simulink model "NarmaMotorS555"  (R2019b)
settings: Solver=FixedStepAuto  StartTime=0.0  StopTime=30  FixedStep=0.001  RelTol=1e-3
libraries: neural x1, simulink x1
settings Model: Creator=Emanuel  LastModifiedBy=Emanuel

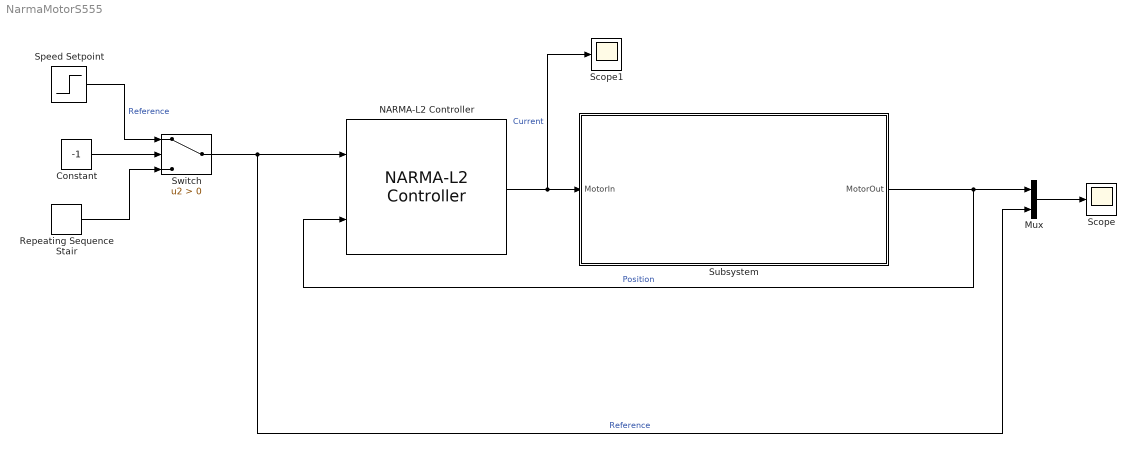
== system NarmaMotorS555 ==
  Constant : Constant  Value=-1
  Mux : Mux  Inputs=2
  NARMA-L2 Controller : neural/Control Systems/NARMA-L2 Controller  Normalize=0  IW1_1=[21.420472575406133586 -21.972703296207392043 -7.9906893081249545929 7.0093970032024079941 8.5373540872644628763 8.8150101640927438496 -2.9213191886093334837 -1.6299775720800899759 -1.2105815169084979122;-0.12814212482981091057 -15.451137614433791967 23.631470507291648886 8.1296696368918119902 -15.652038067620965833 46.375391110128518335 -18.123857574027180561 2.2201217276273146339 -5.7721001387385229009;0.00011021763309481335483 -2.9231777266735832472e-05 1.0017262420479688574e-05 4.4951441027179193515e-06 -1.3997667040411272311e-05 0.00015970236645007296014 -1.3053492369251622356e-05 -0.00010774931406669859316 -0.00020601444658894911294;-10.80852230598250685 2.9694610081311818561 23.641173482018462693 -8.9374523387581881195 -6.2415329671022758973 -12.804217284426561818 8.9963311782389041582 6.791537241510962275 -12.300046900155798824;-2.5462998703491250829 0.40736130073714715838 -18.235100932779950256 1.6768821975697136839 20.314826651060510443 8.341267777448827303 31.645810426981082486 20.102565537518792382 -8.4636642447471075457]  IW3_2=[26.518110030274044675 11.942738916641486568 5.9317929528543604789 -12.906642684649902719 -35.475911845893101315 -0.11447224640092470982 1.1036063891538443471 1.2539998649502879235 1.9551365056904561612;-39.675892314256245186 -12.346459002706955843 12.885795078472623842 15.915516809313654534 24.244911915898089916 -3.9565933976663298921 -13.490028317496282284 -1.9222873594971927602 1.9450222464410471535;-0.49775896817409004402 -20.203686361997281296 15.185910851212808481 6.5982122964106935115 -3.3039127819307578804 5.661531661101603774 1.0333906568373585344 3.2167073441307101334 2.3975065135655868609;-18.741605900013510677 17.739672652356080818 -8.5348038689952723246 -1.7678605588439249008 10.151016666991511173 6.010383209140059968 3.0879575435889647927 6.4865290493294747165 -2.8848587536067671344;9.4392585237701105427 8.6634826964493463208 5.7064818124290734858 4.3740389144362650242 4.6910020487183228255 0.25543532051108375214 0.37978770358499319704 0.25144757086620406206 -0.19880708237697139462]  IW5_3=-3.3096476108531893701  LW2_1=[-33.532867616268568156 -0.062278984235911556688 -126.85135625090671851 -0.22775640561207807777 0.011587551941983549944]  LW4_3=[-0.12271840530871241937 0.019979545310268350539 3.9480102969725656692 -3.8012667565729301167 -4.8370809941710657398]  LW5_4=0.32653514050989068673  LW6_5=0.51420792674405046974  LW6_2=-96.852303453609138728  B1=[2.427680381206728466;-3.6329489870410958119;-0.54248700650812542445;-2.1490981445194363708;1.4125184441117009104]  B2=-34.159715705337887925  B3=[5.6421171826928011583;-1.3367611274533106602;0.50921321783681250395;-3.4202773292942754146;2.3122705363903719444]  B4=-5.5660771533707817937  Limit_output=0  min_output=-Inf  max_output=Inf  Use_Previous_Weights=1  Ts=0.05  S1=5  Ni=5  Nj=5  sim_file=SoleModelNoDistrubance  trainfun=trainlm  Use_validation=1  Use_Testing=1  max_i=40  min_i=1  max_i_int=4  min_i_int=2  sam_training=10000  epochs=100  minp=1.2838861864609374397  maxp=39.753006491435613157  mint=2000.3866487334141766  maxt=39.753006491435613157
      settings: SourceProductName=Deep Learning Toolbox  SourceProductBaseCode=NN
  Repeating Sequence Stair : simulink/Sources/Repeating Sequence Stair  OutValues=[1000 2000 3000 4000 5000].'  tsamp=4  OutMin=[]  OutMax=[]  OutDataTypeStr=double  OutputDataTypeScalingMode=double  OutDataType=fixdt(0,8)  ConRadixGroup=Best Precision: Vector-wise  OutScaling=2^-12
  Scope : Scope
  Scope1 : Scope
  Speed Setpoint : Step  Time=5  Before=2000  After=3000  SampleTime=0
  Subsystem : Subsystem
  Switch : Switch  Criteria=u2 > Threshold
  wires:
  NARMA-L2 Controller/1 -> Scope1/1, Subsystem/1(MotorIn)  "Current"
  Subsystem/1("MotorOut ") -> NARMA-L2 Controller/2, Mux/1  "Position"
  Mux/1 -> Scope/1
  Switch/1 -> Mux/2, NARMA-L2 Controller/1  "Reference"
  Repeating Sequence Stair/1 -> Switch/3
  Speed Setpoint/1 -> Switch/1  "Reference"
  Constant/1 -> Switch/2

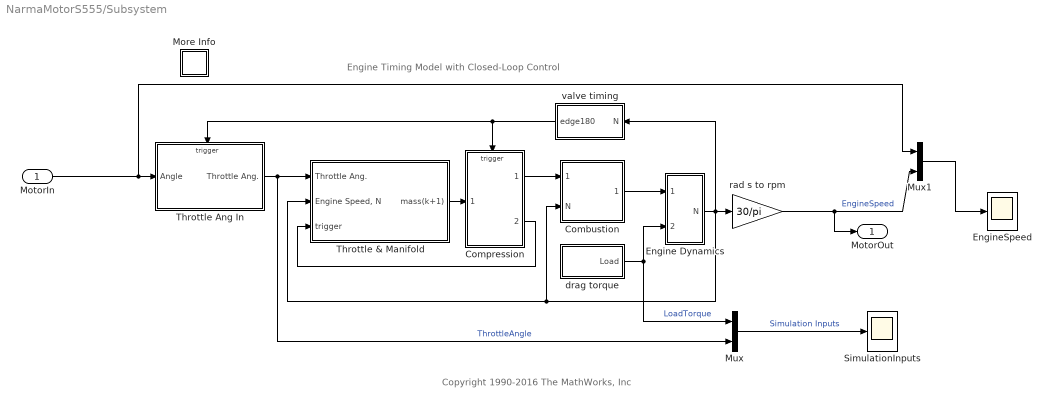
== system NarmaMotorS555/Subsystem ==
  note: Copyright 1990-2016 The MathWorks, Inc
  note: Engine Timing Model with Closed-Loop Control
  MotorIn : Inport
  Combustion : Subsystem
  Compression : Subsystem  TreatAsAtomicUnit=on
  Engine Dynamics : Subsystem
  EngineSpeed : Scope
  More Info : Subsystem
      settings: OpenFcn=showdemo(bdroot(gcb))
      mask Display: disp('?')
  Mux : Mux  Inputs=2
  Mux1 : Mux  Inputs=2
  SimulationInputs : Scope
  Throttle & Manifold : Subsystem
  Throttle Ang In : Subsystem  TreatAsAtomicUnit=on
  drag torque : Subsystem
  rad s to rpm : Gain  Gain=30/pi  SaturateOnIntegerOverflow=on  OutDataTypeStr=Inherit: Same as input  ParamDataTypeStr=Inherit: Same as input
  valve timing : Subsystem
  "MotorOut " : Outport
  wires:
  Combustion/1(Torque) -> Engine Dynamics/1(Teng)
  Throttle Ang In/1(Throttle Ang.) -> Mux/2, Throttle & Manifold/1(Throttle Ang.)  "ThrottleAngle"
  drag torque/1(Load) -> Mux/1, Engine Dynamics/2(Tload)  "LoadTorque"
  MotorIn/1 -> Mux1/1, Throttle Ang In/1(Angle)
  Throttle & Manifold/1(mass(k+1)) -> Compression/1(mass(k+1))
  Compression/2(trigger) -> Throttle & Manifold/3(trigger)
  Mux/1 -> SimulationInputs/1  "Simulation Inputs"
  rad s to rpm/1 -> "MotorOut "/1, Mux1/2  "EngineSpeed"
  Compression/1(mass(k)) -> Combustion/1(Air Charge)
  Mux1/1 -> EngineSpeed/1
  valve timing/1(edge180) -> Throttle Ang In/Trigger, Compression/Trigger
  Engine Dynamics/1(N) -> rad s to rpm/1, valve timing/1(N), Throttle & Manifold/2("Engine Speed, N"), Combustion/2(N)

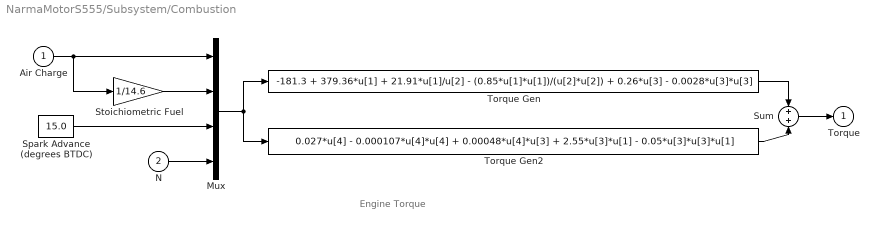
== system NarmaMotorS555/Subsystem/Combustion ==
  note: Engine Torque
  Air Charge : Inport
  N : Inport  Port=2
  Mux : Mux
  Spark Advance (degrees BTDC) : Constant  Value=15.0
  Stoichiometric Fuel : Gain  Gain=1/14.6  SaturateOnIntegerOverflow=on  OutDataTypeStr=Inherit: Same as input  ParamDataTypeStr=Inherit: Same as input
  Sum : Sum  SaturateOnIntegerOverflow=on  InputSameDT=on  OutDataTypeStr=Inherit: Same as first input
  Torque Gen : Fcn  Expr=-181.3 + 379.36*u[1] + 21.91*u[1]/u[2] - (0.85*u[1]*u[1])/(u[2]*u[2]) + 0.26*u[3] - 0.0028*u[3]*u[3]
  Torque Gen2 : Fcn  Expr=0.027*u[4] - 0.000107*u[4]*u[4] + 0.00048*u[4]*u[3] + 2.55*u[3]*u[1] - 0.05*u[3]*u[3]*u[1]
  Torque : Outport  InitialOutput=0
  wires:
  Stoichiometric Fuel/1 -> Mux/2
  Spark Advance (degrees BTDC)/1 -> Mux/3
  N/1 -> Mux/4
  Air Charge/1 -> Stoichiometric Fuel/1, Mux/1
  Mux/1 -> Torque Gen/1, Torque Gen2/1
  Torque Gen2/1 -> Sum/2
  Torque Gen/1 -> Sum/1
  Sum/1 -> Torque/1

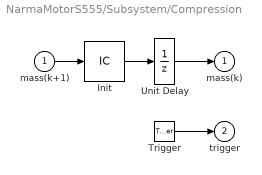
== system NarmaMotorS555/Subsystem/Compression ==
  mass(k+1) : Inport
  Trigger : TriggerPort  TriggerType=either  VariantControl=Variant  ShowOutputPort=on
  Init : InitialCondition  Value=0.152
  Unit Delay : UnitDelay  InitialCondition=0.152  SampleTime=-1  HasFrameUpgradeWarning=on
  mass(k) : Outport  InitialOutput=0.152
  trigger : Outport  Port=2  InitialOutput=-1
  wires:
  Init/1 -> Unit Delay/1
  mass(k+1)/1 -> Init/1
  Unit Delay/1 -> mass(k)/1
  Trigger/1 -> trigger/1

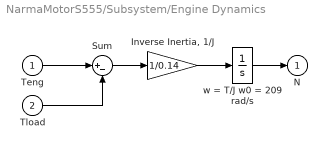
== system NarmaMotorS555/Subsystem/Engine Dynamics ==
  Teng : Inport
  Tload : Inport  Port=2
  "Inverse Inertia, 1/J" : Gain  Gain=1/0.14  SaturateOnIntegerOverflow=on  OutDataTypeStr=Inherit: Same as input  ParamDataTypeStr=Inherit: Same as input
  Sum : Sum  Inputs=|+-  SaturateOnIntegerOverflow=on  InputSameDT=on  OutDataTypeStr=Inherit: Same as first input
  w = T/J w0 = 209 rad/s : Integrator  InitialCondition=209.48
  N : Outport  InitialOutput=0
  wires:
  "Inverse Inertia, 1/J"/1 -> w = T/J w0 = 209 rad/s/1
  w = T/J w0 = 209 rad/s/1 -> N/1
  Sum/1 -> "Inverse Inertia, 1/J"/1
  Teng/1 -> Sum/1
  Tload/1 -> Sum/2

== system NarmaMotorS555/Subsystem/More Info ==

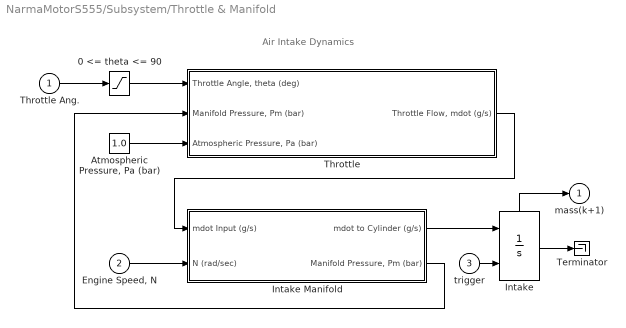
== system NarmaMotorS555/Subsystem/Throttle & Manifold ==
  note: Air Intake Dynamics
  Throttle Ang. : Inport
  "Engine Speed, N" : Inport  Port=2
  trigger : Inport  Port=3
  0 <= theta <= 90 : Saturate  UpperLimit=90  LowerLimit=0
  "Atmospheric Pressure, Pa (bar)" : Constant  Value=1.0
  Intake : Integrator  ExternalReset=either  ShowStatePort=on
  Intake Manifold : Subsystem
  Terminator : Terminator
  Throttle : Subsystem
  mass(k+1) : Outport  InitialOutput=0
  wires:
  0 <= theta <= 90/1 -> Throttle/1("Throttle Angle, theta (deg)")
  Throttle Ang./1 -> 0 <= theta <= 90/1
  Throttle/1("Throttle Flow, mdot (g/s)") -> Intake Manifold/1(mdot Input (g/s))
  "Engine Speed, N"/1 -> Intake Manifold/2(N (rad/sec))
  Intake Manifold/2("Manifold Pressure, Pm (bar)") -> Throttle/2("Manifold Pressure, Pm (bar)")
  Intake Manifold/1(mdot to Cylinder (g/s)) -> Intake/1
  "Atmospheric Pressure, Pa (bar)"/1 -> Throttle/3("Atmospheric Pressure, Pa (bar) ")
  Intake/State -> mass(k+1)/1
  trigger/1 -> Intake/2
  Intake/1 -> Terminator/1

== system NarmaMotorS555/Subsystem/Throttle Ang In ==
  note: Controller Subsystem
  Angle : Inport
  Trigger : TriggerPort  TriggerType=either  VariantControl=Variant
  Throttle Ang. : Outport  InitialOutput=8.973
  wires:
  Angle/1 -> Throttle Ang./1

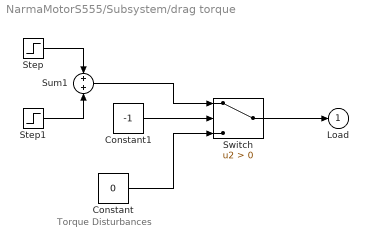
== system NarmaMotorS555/Subsystem/drag torque ==
  note: Torque Disturbances
  Constant : Constant  Value=0
  Constant1 : Constant  Value=-1
  Step : Step  Time=2  Before=25  After=20  SampleTime=0
  Step1 : Step  Time=8  After=5  SampleTime=0
  Sum1 : Sum  SaturateOnIntegerOverflow=on  InputSameDT=on  OutDataTypeStr=Inherit: Same as first input
  Switch : Switch  Criteria=u2 > Threshold
  Load : Outport  InitialOutput=0
  wires:
  Sum1/1 -> Switch/1
  Step/1 -> Sum1/1
  Step1/1 -> Sum1/2
  Switch/1 -> Load/1
  Constant/1 -> Switch/3
  Constant1/1 -> Switch/2

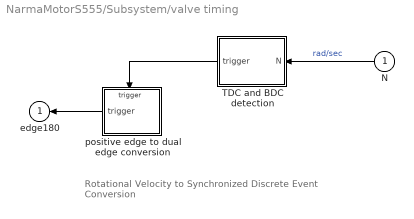
== system NarmaMotorS555/Subsystem/valve timing ==
  note: Rotational Velocity to Synchronized
      | Discrete Event Conversion
  N : Inport
  TDC and BDC detection : Subsystem
  positive edge to dual edge conversion : Subsystem  TreatAsAtomicUnit=on
  edge180 : Outport  InitialOutput=-1
  wires:
  TDC and BDC detection/1(trigger) -> positive edge to dual edge conversion/Trigger
  positive edge to dual edge conversion/1(trigger) -> edge180/1
  N/1 -> TDC and BDC detection/1(N)  "rad/sec"

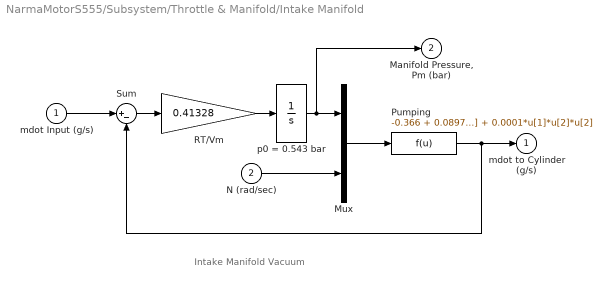
== system NarmaMotorS555/Subsystem/Throttle & Manifold/Intake Manifold ==
  note: Intake Manifold Vacuum
  mdot Input (g/s) : Inport
  N (rad/sec) : Inport  Port=2
  Mux : Mux  Inputs=2
  Pumping : Fcn  Expr=-0.366 + 0.08979*u[1]*u[2] - 0.0337*u[2]*u[1]*u[1] + 0.0001*u[1]*u[2]*u[2]
  RT/Vm : Gain  Gain=0.41328  SaturateOnIntegerOverflow=on  OutDataTypeStr=Inherit: Same as input  ParamDataTypeStr=Inherit: Same as input
  Sum : Sum  Inputs=|+-  SaturateOnIntegerOverflow=on  InputSameDT=on  OutDataTypeStr=Inherit: Same as first input
  p0 = 0.543 bar : Integrator  InitialCondition=.543
  mdot to Cylinder (g/s) : Outport  InitialOutput=0
  "Manifold Pressure, Pm (bar)" : Outport  Port=2  InitialOutput=0
  wires:
  mdot Input (g/s)/1 -> Sum/1
  RT/Vm/1 -> p0 = 0.543 bar/1
  N (rad/sec)/1 -> Mux/2
  Mux/1 -> Pumping/1
  p0 = 0.543 bar/1 -> Mux/1, "Manifold Pressure, Pm (bar)"/1
  Sum/1 -> RT/Vm/1
  Pumping/1 -> Sum/2, mdot to Cylinder (g/s)/1

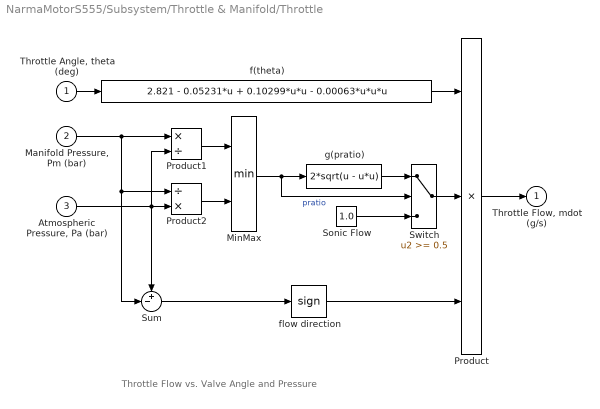
== system NarmaMotorS555/Subsystem/Throttle & Manifold/Throttle ==
  note: Throttle Flow vs. Valve Angle and Pressure
  "Throttle Angle, theta (deg)" : Inport
  "Manifold Pressure, Pm (bar)" : Inport  Port=2
  "Atmospheric Pressure, Pa (bar) " : Inport  Port=3
  MinMax : MinMax  Inputs=2  SaturateOnIntegerOverflow=on  InputSameDT=on
  Product : Product  Inputs=3  SaturateOnIntegerOverflow=on  RndMeth=Zero  InputSameDT=on  OutDataTypeStr=Inherit: Same as first input
  Product1 : Product  Inputs=*/  SaturateOnIntegerOverflow=on  RndMeth=Zero  InputSameDT=on  OutDataTypeStr=Inherit: Same as first input
  Product2 : Product  Inputs=/*  SaturateOnIntegerOverflow=on  RndMeth=Zero  InputSameDT=on  OutDataTypeStr=Inherit: Same as first input
  "Sonic Flow " : Constant  Value=1.0
  Sum : Sum  Inputs=+-|  SaturateOnIntegerOverflow=on  InputSameDT=on  OutDataTypeStr=Inherit: Same as first input
  Switch : Switch  Threshold=0.5  SaturateOnIntegerOverflow=on  InputSameDT=on
  f(theta) : Fcn  Expr=2.821 - 0.05231*u + 0.10299*u*u - 0.00063*u*u*u
  flow direction : Signum
  g(pratio) : Fcn  Expr=2*sqrt(u - u*u)
  "Throttle Flow, mdot (g/s)" : Outport  InitialOutput=0
  wires:
  "Manifold Pressure, Pm (bar)"/1 -> Sum/2, Product2/1, Product1/1
  Product2/1 -> MinMax/2
  Product1/1 -> MinMax/1
  "Atmospheric Pressure, Pa (bar) "/1 -> Sum/1, Product2/2, Product1/2
  g(pratio)/1 -> Switch/1
  "Sonic Flow "/1 -> Switch/3
  Switch/1 -> Product/2
  flow direction/1 -> Product/3
  Sum/1 -> flow direction/1
  MinMax/1 -> Switch/2, g(pratio)/1  "pratio"
  "Throttle Angle, theta (deg)"/1 -> f(theta)/1
  Product/1 -> "Throttle Flow, mdot (g/s)"/1
  f(theta)/1 -> Product/1

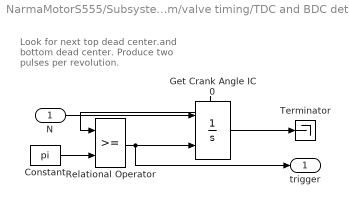
== system NarmaMotorS555/Subsystem/valve timing/TDC and BDC detection ==
  note: Look for next top dead center.and
      | bottom dead center.
      | Produce two pulses per revolution.
  N : Inport
  Constant : Constant  Value=pi
  Get Crank Angle IC 0 : Integrator  ExternalReset=rising  ShowStatePort=on
  Relational Operator : RelationalOperator  OutDataTypeStr=boolean  RndMeth=Nearest  InputSameDT=on
  Terminator : Terminator
  trigger : Outport  InitialOutput=0
  wires:
  N/1 -> Get Crank Angle IC 0/1
  Relational Operator/1 -> trigger/1, Get Crank Angle IC 0/2
  Constant/1 -> Relational Operator/2
  Get Crank Angle IC 0/State -> Relational Operator/1
  Get Crank Angle IC 0/1 -> Terminator/1

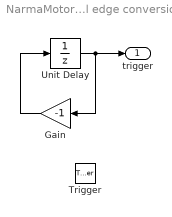
== system NarmaMotorS555/Subsystem/valve timing/positive edge to dual edge conversion ==
  Trigger : TriggerPort  VariantControl=Variant
  Gain : Gain  Gain=-1  SaturateOnIntegerOverflow=on  OutDataTypeStr=Inherit: Same as input  ParamDataTypeStr=Inherit: Same as input
  Unit Delay : UnitDelay  InitialCondition=1  SampleTime=-1  HasFrameUpgradeWarning=on
  trigger : Outport  InitialOutput=-1
  wires:
  Gain/1 -> Unit Delay/1
  Unit Delay/1 -> trigger/1, Gain/1
